simulink library "csu_gml_guidance_mode_logic_lib"  (R2015b)
settings: Solver=ode45  StartTime=0.0  StopTime=10.0  RelTol=1e-3
libraries: util_common_lib x15, util_info_lib x1
settings Model: Creator=Nilesh  LastModifiedBy=Mark Agbayani
settings DataIOCC: SaveFormat=Array
settings DebuggingCC: UnderspecifiedInitializationDetection=Classic  MergeDetectMultiDrivingBlocksExec=none  SolverPrmCheckMsg=warning  StateNameClashWarn=warning
settings HardwareCC: ProdBitPerPointer=32  ProdLargestAtomicFloat=None  ProdIntDivRoundTo=Undefined  ProdEndianess=Unspecified  ProdWordSize=32  ProdHWDeviceType=32-bit Generic
settings GRTTargetCC: GeneratePreprocessorConditionals=Disable all
settings ConfigComp: CovModelRefEnable=Off  CovSFcnEnable=off

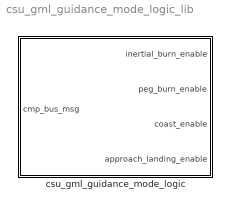
== system csu_gml_guidance_mode_logic_lib ==
  csu_gml_guidance_mode_logic : Subsystem  TreatAsAtomicUnit=on

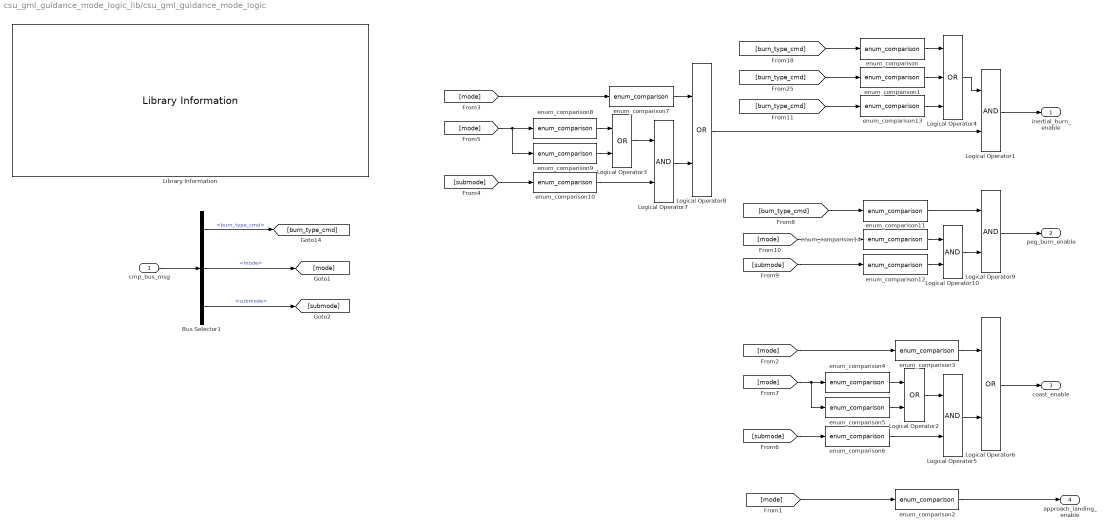
== system csu_gml_guidance_mode_logic_lib/csu_gml_guidance_mode_logic ==
  cmp_bus_msg : Inport
  Bus Selector1 : BusSelector  OutputSignals=burn_type_cmd,mode,submode
  Library Information : util_info_lib/Library Information  owner='jkaidy'
  Logical Operator{1,5,7,9..10} (5 alike) : Logic  AllPortsSameDT=off  OutDataTypeStr=boolean
  Logical Operator{2..3,6,8} (4 alike) : Logic  Operator=OR  AllPortsSameDT=off  OutDataTypeStr=boolean
  Logical Operator4 : Logic  Operator=OR  Inputs=3  AllPortsSameDT=off  OutDataTypeStr=boolean
  enum_comparison{,1..5,7..14} (14 alike) : util_common_lib/enum_comparison  comparison_type===
  enum_comparison6 : util_common_lib/enum_comparison  comparison_type=~=
  inertial_burn_enable : Outport
  peg_burn_enable : Outport  Port=2
  coast_enable : Outport  Port=3
  approach_landing_enable : Outport  Port=4
  wires:
  enum_comparison13/1 -> Logical Operator4/3
  [burn_type_cmd] -> enum_comparison13/1
  enum_comparison11/1 -> Logical Operator9/1
  Logical Operator10/1 -> Logical Operator9/2
  enum_comparison14/1 -> Logical Operator10/1
  enum_comparison12/1 -> Logical Operator10/2
  Logical Operator8/1 -> Logical Operator1/2
  Logical Operator7/1 -> Logical Operator8/2
  enum_comparison7/1 -> Logical Operator8/1
  enum_comparison10/1 -> Logical Operator7/2
  Logical Operator3/1 -> Logical Operator7/1
  enum_comparison9/1 -> Logical Operator3/2
  enum_comparison8/1 -> Logical Operator3/1
  [submode] -> enum_comparison10/1
  [mode] -> enum_comparison8/1, enum_comparison9/1
  [mode] -> enum_comparison7/1
  Logical Operator6/1 -> coast_enable/1
  Logical Operator5/1 -> Logical Operator6/2
  enum_comparison3/1 -> Logical Operator6/1
  enum_comparison6/1 -> Logical Operator5/2
  Logical Operator2/1 -> Logical Operator5/1
  enum_comparison5/1 -> Logical Operator2/2
  enum_comparison4/1 -> Logical Operator2/1
  [submode] -> enum_comparison6/1
  [mode] -> enum_comparison4/1, enum_comparison5/1
  [mode] -> enum_comparison3/1
  Bus Selector1/3 -> [submode]  "<submode>"
  Bus Selector1/2 -> [mode]  "<mode>"
  [burn_type_cmd] -> enum_comparison1/1
  [burn_type_cmd] -> enum_comparison/1
  Logical Operator4/1 -> Logical Operator1/1
  enum_comparison1/1 -> Logical Operator4/2
  enum_comparison/1 -> Logical Operator4/1
  enum_comparison2/1 -> approach_landing_enable/1
  [mode] -> enum_comparison2/1
  Logical Operator1/1 -> inertial_burn_enable/1
  cmp_bus_msg/1 -> Bus Selector1/1
  Bus Selector1/1 -> [burn_type_cmd]  "<burn_type_cmd>"
  [burn_type_cmd] -> enum_comparison11/1
  Logical Operator9/1 -> peg_burn_enable/1
  [submode] -> enum_comparison12/1
  [mode] -> enum_comparison14/1
